simulink model "s0415"  (Simulink 7.0)
settings: Solver=ode3  SolverMode=SingleTasking  StartTime=0.0  StopTime=10  FixedStep=1  MaxStep=1  RelTol=1e-3  AbsTol=1e-6
values from neighbouring files (symbols this model uses):
  Kpr = 10    [m0108d.m]    (also in m0109b.m = 1; m0113c.m; m0404Bsp.m = 3)
undefined symbols (not defined in the file or in its folder): edach, Kir, TB, ymax, ymin
settings Model: Creator=froriep  LastModifiedBy=froriep
settings DataIOCC: LimitDataPoints=off  SaveOutput=off  TimeSaveName=t
settings OptimizationCC: BooleanDataType=off  InlineInvariantSignals=on
settings DebuggingCC: SaveWithParameterizedLinksMsg=none  SignalResolutionControl=TryResolveAllWithWarning  SolverPrmCheckMsg=none  MultiTaskDSMMsg=warning  MultiTaskCondExecSysMsg=none  StrictBusMsg=None
settings HardwareCC: TargetUnknown=on
settings RTWCC: IncludeERTFirstTime=on
settings GRTTargetCC: TargetFcnLib=ansi_tfl_tmw.mat  ModelReferenceCompliant=off  CompOptLevelCompliant=off  MatFileLogging=off

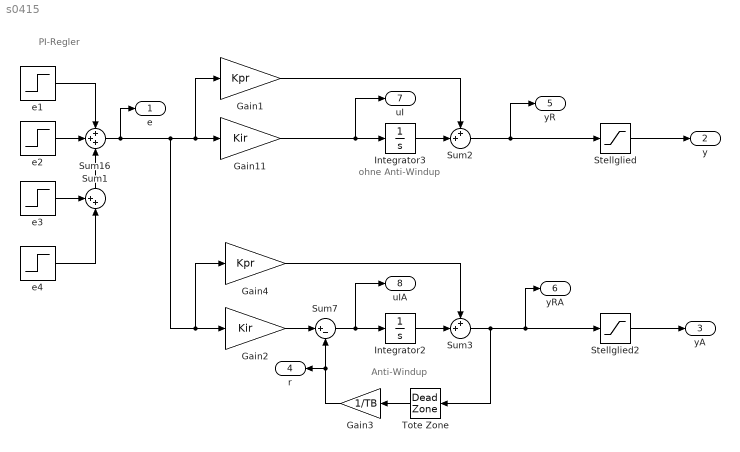
== system s0415 ==
  note: PI-Regler
  note: Anti-Windup
  note: ohne Anti-Windup
  Gain1 : Gain  Gain=Kpr  ParameterDataType=sfix(16)  ParameterScaling=2^0  OutDataType=sfix(16)  OutScaling=2^0
  Gain11 : Gain  Gain=Kir  ParameterDataType=sfix(16)  ParameterScaling=2^0  OutDataType=sfix(16)  OutScaling=2^0
  Gain2 : Gain  Gain=Kir  ParameterDataType=sfix(16)  ParameterScaling=2^0  OutDataType=sfix(16)  OutScaling=2^0
  Gain3 : Gain  Orientation=left  Gain=1/TB  ParameterDataType=sfix(16)  ParameterScaling=2^0  OutDataType=sfix(16)  OutScaling=2^0
  Gain4 : Gain  Gain=Kpr  ParameterDataType=sfix(16)  ParameterScaling=2^0  OutDataType=sfix(16)  OutScaling=2^0
  Integrator2 : Integrator
  Integrator3 : Integrator
  Stellglied : Saturate  UpperLimit=ymax  LowerLimit=ymin  OutDataType=sfix(16)  OutScaling=2^0
  Stellglied2 : Saturate  UpperLimit=ymax  LowerLimit=ymin  OutDataType=sfix(16)  OutScaling=2^0
  Sum1 : Sum  Orientation=up  Inputs=++|  OutDataType=sfix(16)  OutScaling=2^0
  Sum16 : Sum  Inputs=+++  OutDataType=sfix(16)  OutScaling=2^0
  Sum2 : Sum  Inputs=++|  OutDataType=sfix(16)  OutScaling=2^0
  Sum3 : Sum  Inputs=++|  OutDataType=sfix(16)  OutScaling=2^0
  Sum7 : Sum  Inputs=|+-  OutDataType=sfix(16)  OutScaling=2^0  SaturateOnIntegerOverflow=on  InputSameDT=on
  Tote Zone : DeadZone  Orientation=left  LowerValue=ymin  UpperValue=ymax  SaturateOnIntegerOverflow=on
  e1 : Step  Time=.1  After=edach  SampleTime=0
  e2 : Step  Time=10  After=-0.5*edach  SampleTime=0
  e3 : Step  Time=15  After=-0.5*edach  SampleTime=0
  e4 : Step  Time=20  After=-edach  SampleTime=0
  e : Outport  OutDataType=sfix(16)  OutScaling=2^0
  y : Outport  Port=2  OutDataType=sfix(16)  OutScaling=2^0
  yA : Outport  Port=3  OutDataType=sfix(16)  OutScaling=2^0
  r : Outport  Orientation=left  Port=4  OutDataType=sfix(16)  OutScaling=2^0
  yR : Outport  Port=5  OutDataType=sfix(16)  OutScaling=2^0
  yRA : Outport  Port=6  OutDataType=sfix(16)  OutScaling=2^0
  uI : Outport  Port=7  OutDataType=sfix(16)  OutScaling=2^0
  uIA : Outport  Port=8  OutDataType=sfix(16)  OutScaling=2^0
  wires:
  Gain11/1 -> Integrator3/1, uI/1
  Gain2/1 -> Sum7/1
  Sum7/1 -> Integrator2/1, uIA/1
  Tote Zone/1 -> Gain3/1
  Gain3/1 -> Sum7/2, r/1
  Stellglied2/1 -> yA/1
  Stellglied/1 -> y/1
  e1/1 -> Sum16/1
  e2/1 -> Sum16/2
  Sum16/1 -> Gain11/1, Gain1/1, Gain2/1, Gain4/1, e/1
  e3/1 -> Sum1/1
  Sum1/1 -> Sum16/3
  e4/1 -> Sum1/2
  Gain1/1 -> Sum2/1
  Integrator3/1 -> Sum2/2
  Sum2/1 -> Stellglied/1, yR/1
  Integrator2/1 -> Sum3/2
  Sum3/1 -> Tote Zone/1, Stellglied2/1, yRA/1
  Gain4/1 -> Sum3/1
